simulink model "pompa"  (R2023b)
settings: Solver=VariableStepAuto  StartTime=0.0  StopTime=10.0  RelTol=1e-3
values from neighbouring files (symbols this model uses):
  k11 = k2^2+4*(k-k3)*k1    (= 0.0933546)    [untitled2.m]
  k12 = 8*(k-k3)    (= 0.2848)    [untitled2.m]
  k13 = 2*(k-k3)    (= 0.0712)    [untitled2.m]
  k2 = -0.015    [untitled2.m]
settings Model: Creator=diana.forrai  LastModifiedBy=diana.forrai

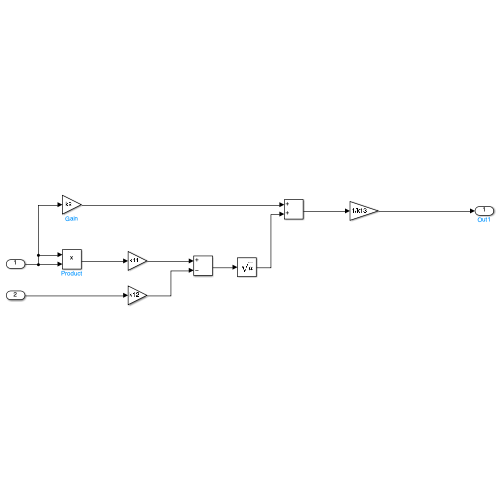
[thumbnail: Simulink's stored preview of the top-level diagram]
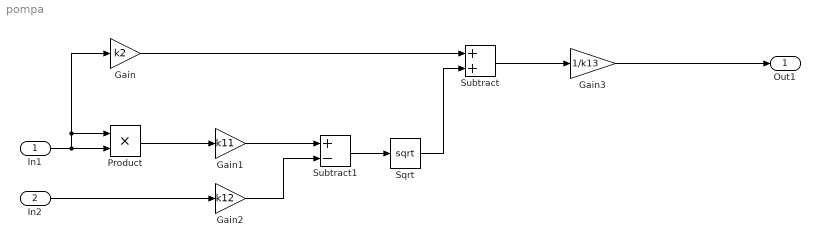
== system pompa ==
  In1 : Inport
  In2 : Inport  Port=2
  Gain : Gain  Gain=k2
  Gain1 : Gain  Gain=k11
  Gain2 : Gain  Gain=k12
  Gain3 : Gain  Gain=1/k13
  Product : Product
  Sqrt : Sqrt
  Subtract : Sum
  Subtract1 : Sum  Inputs=+-
  Out1 : Outport
  wires:
  Subtract/1 -> Gain3/1
  Gain/1 -> Subtract/1
  In1/1 -> Product/1, Gain/1, Product/2
  Product/1 -> Gain1/1
  Gain1/1 -> Subtract1/1
  Subtract1/1 -> Sqrt/1
  Sqrt/1 -> Subtract/2
  Gain2/1 -> Subtract1/2
  In2/1 -> Gain2/1
  Gain3/1 -> Out1/1
